simulink model "ident_sin_real"  (R2018b)
settings: Solver=ode5  StartTime=0.0  StopTime=simtime  FixedStep=Ts  RelTol=1e-3  EnableMultiTasking=on
values from neighbouring files (symbols this model uses):
  freq = 0.01    [incercare1.m]    (also in incercare2.m)
  M = amp_max - scale    [incercare1.m]    (also in incercare2.m)
  Phi = freq*2*pi*(525.238 - 527.813)    (= -0.16179202166)    [incercare1.m]    (also in incercare2.m)
  Ts = mean(diff(t))    [incercare1.m]    (also in incercare2.m; sin_0185.mat = 0.005)
settings Model: Creator=Marcian  LastModifiedBy=Marcian

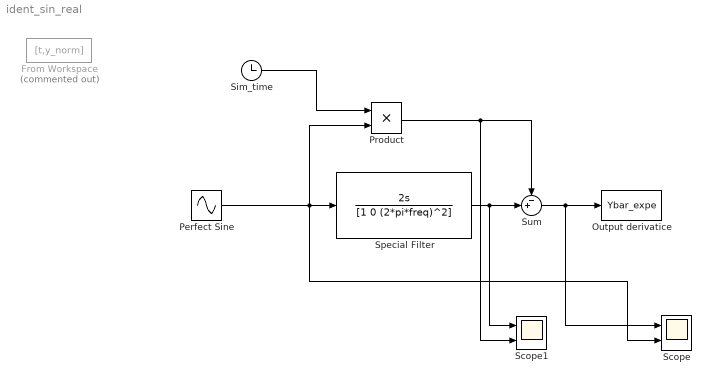
== system ident_sin_real ==
  From Workspace : FromWorkspace  Commented=on  VariableName=[t,y_norm]  SampleTime=Ts
  Output derivatice : ToWorkspace  VariableName=Ybar_expe  SampleTime=Ts
      settings: Save2DSignal=2-D array (concatenate along first dimension)
  Perfect Sine : Sin  Amplitude=M  Frequency=2*pi*freq  Phase=Phi  SampleTime=0
  Product : Product  RndMeth=Zero
  Scope : Scope  NumInputPorts=2
  Scope1 : Scope  NumInputPorts=2
  Sim_time : Clock
      settings: Decimation=5
  Special Filter : TransferFcn  Numerator=[2 0]  Denominator=[1 0 (2*pi*freq)^2]
  Sum : Sum  Inputs=-+|
  wires:
  Sim_time/1 -> Product/1
  Special Filter/1 -> Scope1/1, Sum/2
  Product/1 -> Scope1/2, Sum/1
  Sum/1 -> Output derivatice/1, Scope/1
  Perfect Sine/1 -> Special Filter/1, Scope/2, Product/2
